simulink model "Fig517"  (R2014b)
settings: Solver=ode3  StartTime=0.0  StopTime=0.262144  FixedStep=1e-6  RelTol=1e-3
libraries: commchan3 x1, commseqgen2 x1
settings Model: Creator=Silage  LastModifiedBy=Silage

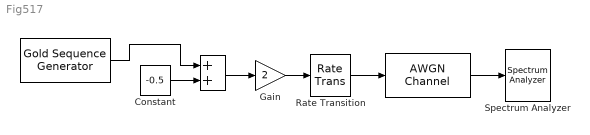
== system Fig517 ==
  " " : commchan3/AWGN Channel  InputProcessing=Columns as channels (frame based)  seed=randseed  noiseMode=Variance from mask  EbNodB=10  EsNodB=10  SNRdB=10  bitsPerSym=1  Ps=1  Tsym=1  variance=1
  "  " : commseqgen2/Gold Sequence Generator  genPoly1=[1 0 0 1 0 1]  iniState1=[1 1 1 0 1]  genPoly2=[1 1 1 1 0 1]  iniState2=[1 0 0 0 1]  index=0  shift=0  outVarSiz=off  maxOutSizeMode=Dialog parameter  maxOutSize=[10 1]  ts=1e-3  frameBased=off  sampPerFrame=1  reset=off  outDataType=double
  "    " : Sum
  Constant : Constant  Value=-0.5
  Gain : Gain  Gain=2
  Rate Transition : RateTransition  OutPortSampleTime=1e-6
  Spectrum Analyzer : SpectrumAnalyzer
  wires:
  "  "/1 -> "    "/1
  Constant/1 -> "    "/2
  "    "/1 -> Gain/1
  " "/1 -> Spectrum Analyzer/1
  Gain/1 -> Rate Transition/1
  Rate Transition/1 -> " "/1
